simulink model "verify_Heat_Capacity2_mdl"  (R2018b)
settings: Solver=ode45  StartTime=0.0  StopTime=5  RelTol=1e-3  EnableMultiTasking=on
libraries: carnot x2, simulink x1
settings Model: Creator=darl  LastModifiedBy=drhf
settings DataIOCC: SaveFormat=Array
settings OptimizationCC: LifeSpan=inf
settings DebuggingCC: SFUnexpectedBacktrackingDiag=warning  SFNoUnconditionalDefaultTransitionDiag=warning  SFExecutionAtInitializationDiag=none
settings HardwareCC: ProdBitPerSizeT=32  ProdBitPerPtrDiffT=32  ProdWordSize=32  ProdHWDeviceType=Specified
settings SFSimCC: SimUseLocalCustomCode=off
settings RTWCC: RTWUseLocalCustomCode=off
settings CodeAppCC: StateflowObjectComments=on
settings GRTTargetCC: TargetLangStandard=C89/C90 (ANSI)
settings ConfigComp: CovMetricSettings=dw  CovHtmlReporting=on  CovSaveCumulativeToWorkspaceVar=on  CovSaveSingleToWorkspaceVar=on  CovExternalEMLEnable=off

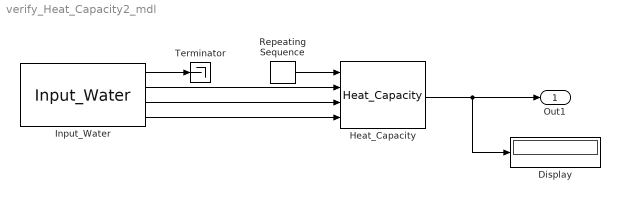
== system verify_Heat_Capacity2_mdl ==
  Display : Display
  Heat_Capacity : carnot/Basic/Material_Properties/Heat_Capacity  VariantControl=CarlibClassic  INPUTARGUMENTS=state variables (classic)  DEBUGLEVEL=DEBUGLEVEL  MAXTOTALWARNINGS=inf  MAXCONSECUTIVEWARNINGS=inf  WRITETOFILE=0  FILENAME='errors.txt'
  Input_Water : carnot/Basic/Material_Properties/Input_Water  T=20  p=2e6  xd=0
  Repeating Sequence : simulink/Sources/Repeating Sequence  rep_seq_t=0:6  rep_seq_y=[0.01 4.44 10 15.6 21.1 26.7 32.2]
  Terminator : Terminator
  Out1 : Outport
  wires:
  Input_Water/4 -> Heat_Capacity/4
  Input_Water/3 -> Heat_Capacity/3
  Input_Water/2 -> Heat_Capacity/2
  Input_Water/1 -> Terminator/1
  Repeating Sequence/1 -> Heat_Capacity/1
  Heat_Capacity/1 -> Display/1, Out1/1
